simulink model "ThermalControl"  (R2023b)
settings: Solver=FixedStepDiscrete  StartTime=0.0  StopTime=10000  FixedStep=0.1  RelTol=1e-3
undefined symbols (not defined in the file): EnvAirTempC, pump, T_set
libraries: slpidlib x1
settings Model: DataDictionary=VirtualVehicleTemplate.sldd  ModifiedByFormat=The MathWorks, Inc.  Creator=The MathWorks, Inc.  LastModifiedBy=The MathWorks, Inc.
settings SolverCC: PositivePriorityOrder=on  AutoInsertRateTranBlk=on

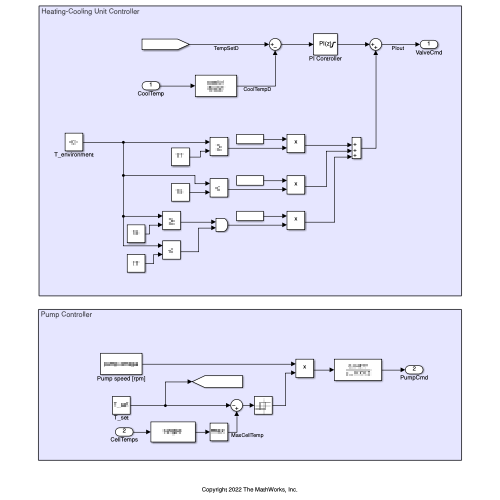
[thumbnail: Simulink's stored preview of the top-level diagram]
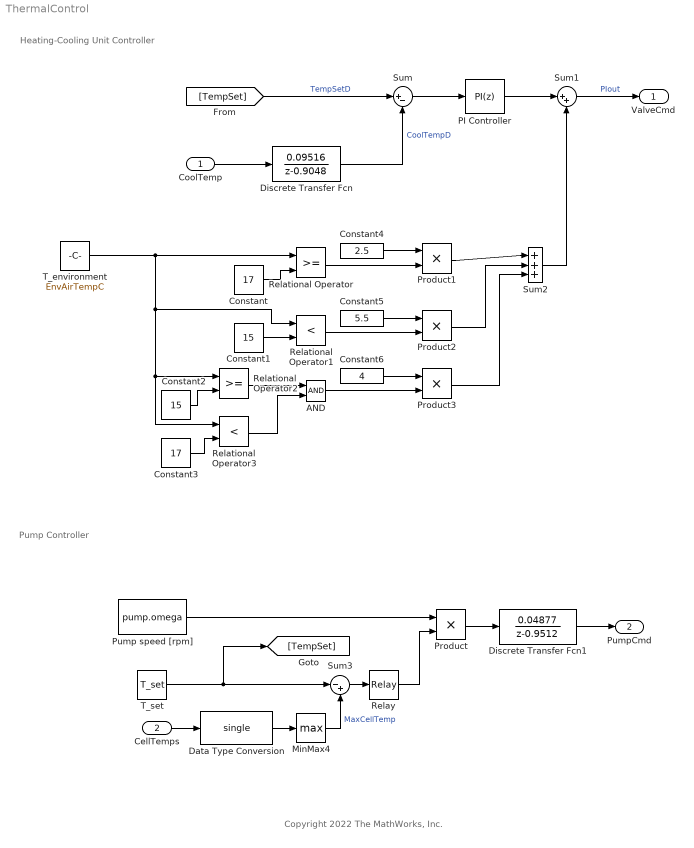
== system ThermalControl ==
  note: Heating-Cooling Unit Controller
  note: Pump Controller
  note: Copyright 2022 The MathWorks, Inc.
  CoolTemp : Inport
  CellTemps : Inport  Port=2  PortDimensions=PlntBattNumCellSer
  AND : Logic  IconShape=distinctive  AllPortsSameDT=off  OutDataTypeStr=boolean
  Constant : Constant  Value=17  SampleTime=-1
  Constant1 : Constant  Value=15  SampleTime=-1
  Constant2 : Constant  Value=15  SampleTime=-1
  Constant3 : Constant  Value=17  SampleTime=-1
  Constant4 : Constant  Value=2.5  SampleTime=-1
  Constant5 : Constant  Value=5.5  SampleTime=-1
  Constant6 : Constant  Value=4  SampleTime=-1
  Data Type Conversion : DataTypeConversion  OutDataTypeStr=single  SaturateOnIntegerOverflow=off  RndMeth=Floor
  Discrete Transfer Fcn : DiscreteTransferFcn  Numerator=[0.09516]  Denominator=[1 -0.9048]  InitialStates=T_set
  Discrete Transfer Fcn1 : DiscreteTransferFcn  Numerator=[0.04877]  Denominator=[1 -0.9512]
  MinMax4 : MinMax  Function=max
  PI Controller : slpidlib/PID Controller  Controller=PI  Form=Parallel  TimeDomain=Discrete-time  UseExternalTs=off  SampleTime=-1  IntegratorMethod=Forward Euler  FilterMethod=Forward Euler  ControllerParametersSource=internal  P=1  I=1  UseKiTs=off  D=0  N=100  UseFilter=on  TunerSelectOption=Transfer Function Based (PID Tuner App)  ZeroCross=off  InitialConditionSource=internal  InitialConditionForIntegrator=0  InitialConditionForFilter=0  DifferentiatorICPrevScaledInput=0  ExternalReset=none  TrackingMode=off  Kt=1  LimitOutput=on  SatLimitsSource=internal  UpperSaturationLimit=2.5  LowerSaturationLimit=-2.5  LinearizeAsGain=on  AntiWindupMode=clamping  Kb=1  LimitIntegrator=off  UpperIntegratorSaturationLimit=inf  LowerIntegratorSaturationLimit=-inf  POutMin=[]  POutMax=[]  IOutMin=[]  IOutMax=[]  DOutMin=[]  DOutMax=[]  NOutMin=[]  NOutMax=[]  SumOutMin=[]  SumOutMax=[]  SaturationOutMin=[]  SaturationOutMax=[]  PParamMin=[]  PParamMax=[]  IParamMin=[]  IParamMax=[]  DParamMin=[]  DParamMax=[]  NParamMin=[]  NParamMax=[]  KbParamMin=[]  KbParamMax=[]  KtParamMin=[]  KtParamMax=[]  KbOutMin=[]  KbOutMax=[]  KtOutMin=[]  KtOutMax=[]  IntegratorOutMin=[]  IntegratorOutMax=[]  FilterOutMin=[]  FilterOutMax=[]  SumI1OutMin=[]  SumI1OutMax=[]  SumI2OutMin=[]  SumI2OutMax=[]  SumI3OutMin=[]  SumI3OutMax=[]  SumI4OutMin=[]  SumI4OutMax=[]  SumDOutMin=[]  SumDOutMax=[]  DifferentiatorOutMin=[]  DifferentiatorOutMax=[]  FilterDiffOutCoefMin=[]  FilterDiffOutCoefMax=[]  ReciprocalOutMin=[]  ReciprocalOutMax=[]  SumDenOutMin=[]  SumDenOutMax=[]  SumNumOutMin=[]  SumNumOutMax=[]  DivideOutMin=[]  DivideOutMax=[]  UdiffTsProdOutMin=[]  UdiffTsProdOutMax=[]  NTsProdOutMin=[]  NTsProdOutMax=[]  UintegralTsProdOutMin=[]  UintegralTsProdOutMax=[]  UngainTsProdOutMin=[]  UngainTsProdOutMax=[]  ClampingZeroOutDataTypeStr=Inherit: Inherit via back propagation  ClampingZeroOutMin=[]  ClampingZeroOutMax=[]  FilterDenConstantOutDataTypeStr=Inherit: Inherit via back propagation  FilterDenConstantOutMin=[]  FilterDenConstantOutMax=[]  PCopyOutDataTypeStr=Inherit: Inherit via back propagation  PCopyOutMin=[]  PCopyOutMax=[]  NCopyOutDataTypeStr=Inherit: Inherit via back propagation  NCopyOutMin=[]  NCopyOutMax=[]  IntegratorContinuousStateAttributes=''  IntegratorStateMustResolveToSignalObject=off  IntegratorRTWStateStorageClass=Auto  FilterContinuousStateAttributes=''  FilterStateMustResolveToSignalObject=off  FilterRTWStateStorageClass=Auto  ParallelPVariant=InternalParameters  IdealPVariant=Disabled  IVariant=InternalParameters  DVariant=Disabled  IntegratorVariant=Discrete  SatVariant=Enabled  AWVariant=DiscClampingParallel  PCopyVariant=Disabled  TRVariant=Disabled  FdbkBlocksVariant=Forward  IdealPFdbkVariant=Disabled  SatFdbkVariant=Disabled  DerivativeFilterVariant=Disabled  NVariant=Disabled  NCopyVariant=Disabled_SignalSpec  FilterICVariant=Disabled  IntegratorICVariant=InternalICs  ExternalResetVariant=Disabled  TRSumVariant=Passthrough  SumFdbkVariant=Disabled  SumVariant=Sum_PI  TsampFilterVariant=InternalTs  TsampNgainVariant=Passthrough  TsampIntegralVariant=Disabled_SignalSpec  ExternalSaturationOutDataTypeStr=Inherit: Same as second input
      settings: LibrarySourceBlock=simulink/Discrete/Discrete PID Controller
  Product{,1..3} (4 alike) : Product
  Pump speed [rpm] : Constant  Value=pump.omega  SampleTime=-1
  Relational Operator : RelationalOperator  OutDataTypeStr=boolean  RndMeth=Simplest  InputSameDT=off
  Relational Operator1 : RelationalOperator  Operator=<  OutDataTypeStr=boolean  RndMeth=Simplest  InputSameDT=off
  Relational Operator2 : RelationalOperator  OutDataTypeStr=boolean  RndMeth=Simplest  InputSameDT=off
  Relational Operator3 : RelationalOperator  Operator=<  OutDataTypeStr=boolean  RndMeth=Simplest  InputSameDT=off
  Relay : Relay  OnSwitchValue=+1  OffSwitchValue=0.1
  Sum : Sum  Inputs=|+-
  Sum1 : Sum  Inputs=|++
  Sum2 : Sum  Inputs=|+++
  Sum3 : Sum  Inputs=|-+
  T_environment : Constant  Value=EnvAirTempC  SampleTime=-1
  T_set : Constant  Value=T_set  SampleTime=-1
  ValveCmd : Outport
  PumpCmd : Outport  Port=2
  wires:
  Constant/1 -> Relational Operator/2
  Product3/1 -> Sum2/3
  Constant1/1 -> Relational Operator1/2
  Relational Operator2/1 -> AND/1
  Constant2/1 -> Relational Operator2/2
  Product2/1 -> Sum2/2
  Relational Operator1/1 -> Product2/2
  T_environment/1 -> Relational Operator1/1, Relational Operator3/1, Relational Operator2/1, Relational Operator/1
  Discrete Transfer Fcn/1 -> Sum/2  "CoolTempD"
  Constant3/1 -> Relational Operator3/2
  Relational Operator/1 -> Product1/2
  AND/1 -> Product3/2
  CoolTemp/1 -> Discrete Transfer Fcn/1
  Relational Operator3/1 -> AND/2
  Sum3/1 -> Relay/1
  CellTemps/1 -> Data Type Conversion/1
  Relay/1 -> Product/2
  Product/1 -> Discrete Transfer Fcn1/1
  Pump speed [rpm]/1 -> Product/1
  MinMax4/1 -> Sum3/2  "MaxCellTemp"
  Data Type Conversion/1 -> MinMax4/1
  Discrete Transfer Fcn1/1 -> PumpCmd/1
  T_set/1 -> [TempSet], Sum3/1
  [TempSet] -> Sum/1  "TempSetD"
  Constant4/1 -> Product1/1
  Constant5/1 -> Product2/1
  Constant6/1 -> Product3/1
  Product1/1 -> Sum2/1
  Sum2/1 -> Sum1/2
  Sum1/1 -> ValveCmd/1  "PIout"
  PI Controller/1 -> Sum1/1
  Sum/1 -> PI Controller/1
